simulink model "Ejercicio_6"  (R2021b)
settings: Solver=VariableStepAuto  StartTime=0.0  StopTime=10.0  RelTol=1e-3
libraries: commrandsrc3 x1, dsparch4 x1
settings Model: Creator=Hagui  LastModifiedBy=Hagui

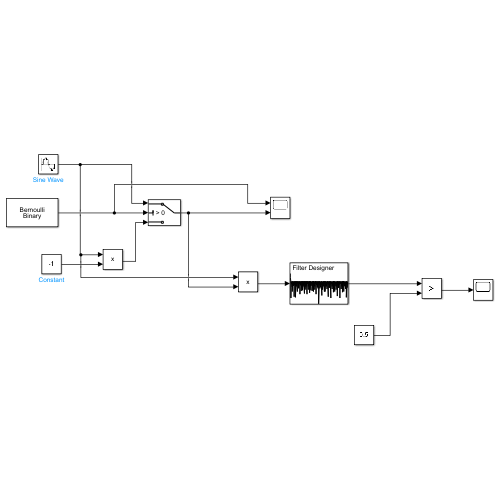
[thumbnail: Simulink's stored preview of the top-level diagram]
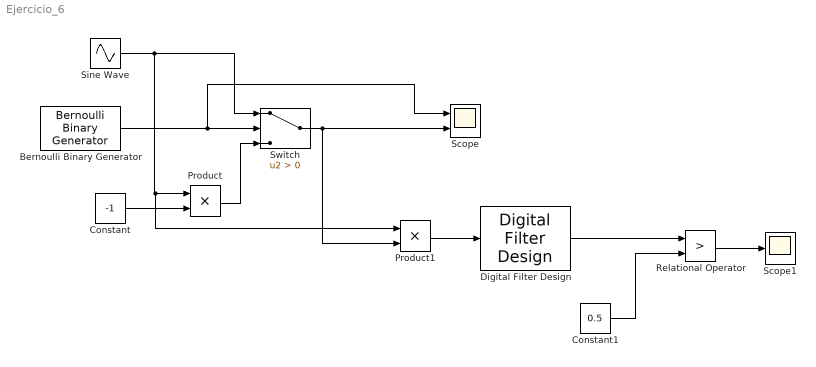
== system Ejercicio_6 ==
  Bernoulli Binary Generator : commrandsrc3/Bernoulli Binary Generator  ProbabilityOfZero=0.5  SeedSource=Auto  Seed=0  SampleTime=1  SamplesPerFrame=1  OutputDataType=double  SimulateUsing=Interpreted execution
  Constant : Constant  Value=-1
  Constant1 : Constant  Value=0.5
  Digital Filter Design : dsparch4/Digital Filter Design  mwdsp_browser_bugfix_var=off
  Product : Product
  Product1 : Product
  Relational Operator : RelationalOperator  Operator=>  OutDataTypeStr=boolean  RndMeth=Simplest
  Scope : Scope  NumInputPorts=2
  Scope1 : Scope
  Sine Wave : Sin  Frequency=4*pi*100  SampleTime=0.0001
  Switch : Switch  Criteria=u2 > Threshold
  wires:
  Bernoulli Binary Generator/1 -> Scope/1, Switch/2
  Sine Wave/1 -> Product1/1, Product/1, Switch/1
  Product/1 -> Switch/3
  Constant/1 -> Product/2
  Switch/1 -> Product1/2, Scope/2
  Digital Filter Design/1 -> Relational Operator/1
  Constant1/1 -> Relational Operator/2
  Relational Operator/1 -> Scope1/1
  Product1/1 -> Digital Filter Design/1
